simulink subsystem "Reefscape_Elevator_Motor_Control_sub"  (R2023b)
settings: Solver=VariableStepAuto  StartTime=0.0  StopTime=10.0  RelTol=1e-3
undefined symbols (not defined in the file): Elevator_Bottom_DC, Elevator_Error_Bottom_Disable, Elevator_Error_Increase, Elevator_Gain_Int, Elevator_Gain_Prop, Elevator_Height_Error_Threshold, Elevator_Height_Lower_Limit_Coral_Arm_Input, Elevator_Height_Lower_Limit_Out, Elevator_Hold_at_Top_DC, Elevator_Int_IC, Elevator_Int_LL, Elevator_Int_UL, Elevator_Total_LL, Elevator_Total_UL
libraries: simulink x6, Controls_Components_lib x1
settings Model: Creator=ander  LastModifiedBy=ander

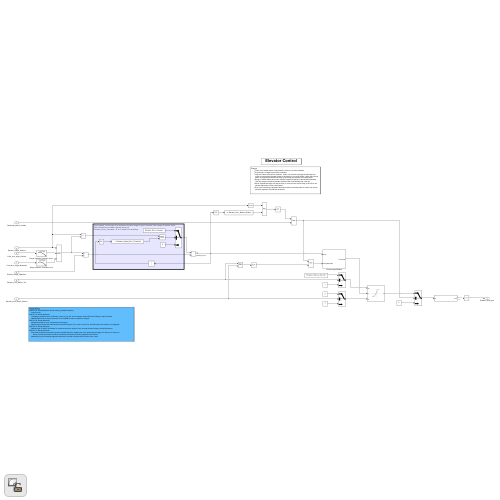
[thumbnail: Simulink's stored preview of the top-level diagram]
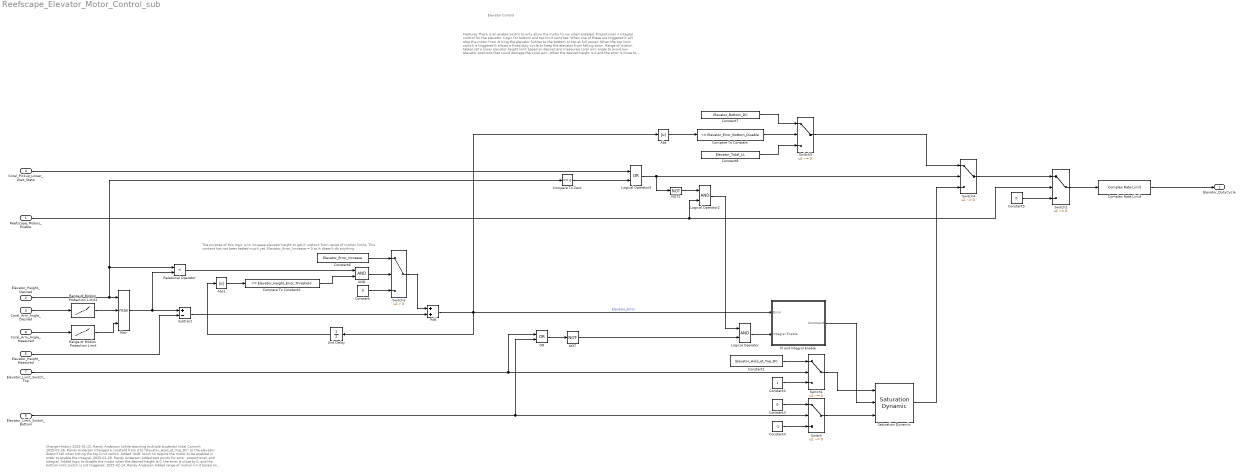
== system Reefscape_Elevator_Motor_Control_sub ==
  note: The purpose of this logic is to increase elevator height to get it unstock from range of motion limits.
      | This content has not been tested much yet.
      | Elevator_Error_Increase = 0 so it doesn't do anything.
  note: Elevator Control
  note: Features
      | There is an enable switch to only allow the motor to run when enabled.
      | Proportional + Integral control for the elevator.
      | Logic for bottom and top limit switches. When one of these are triggered it will stop the motor from driving the elevator further to the bottom or top at full power. When the top limit switch is triggered it allows a fixed duty cycle to keep the elevator from falling down.
      | Range of motion tables set a lower elevator height limit based on desired and measured coral arm angle to avoid low elevator positions that could damage the coral arm.
      | When the desired height is 0 and the error is close to 0 then set the duty cycle to 0 so the elevator falls down to hit the limit switch.
      | Duty cycle increasing magnitude rate limit provides a smoother start of motion from a stop (less jerk applied to mechanical hardware).
  note: Change History
      | 2025-01-22, Randy Anderson (while teaching multiple students)
      | Inital Commit
      | 2025-01-26, Randy Anderson
      | Changed a constant from 0 to 'Elevator_Hold_at_Top_DC' so the elevator doesn't fall when hitting the top limit switch.
      | Added 'AND' block to require the motor to be enabled in order to enable the integral.
      | 2025-01-28, Randy Anderson
      | Added test points for error, proportional, and integral.
      | Added logic to disable the motor when the desired height is 0, the error is close to 0, and the bottom limit switch is not triggered.
      | 2025-02-14, Randy Anderson
      | Added range of motion limit based on measured coral arm angle to force enough elevator height to avoid interference.
      | 2025-02-15, Randy Anderson
      | Removed the bottom limit switch input the the AND block for disabling the motor when desired height is 0 and error is close to 0.
      | When the limit switch was included it resulted in the elevator bouncing up/down off the bottom.
      | Added duty cycle increasing magnitude rate limit to provide smoother start of motion from a stop.
      | 2025-02-24, Randy Anderson
      | Added 'Coral_Pickup_Lower_Wait_State' input.
      | Added a new parameter value to force the elevator down to a fixed duty cycle in some cases.
  Reefscape_Motors_Enable : Inport
  Elevator_Height_Desired : Inport  Port=2
  Coral_Arm_Angle_Desired : Inport  Port=3
  Coral_Pickup_Lower_Wait_State : Inport  Port=4
  Elevator_Height_Measured : Inport  Port=5
  Elevator_Limit_Switch_Bottom : Inport  Port=6
  Elevator_Limit_Switch_Top : Inport  Port=7
  Coral_Arm_Angle_Measured : Inport  Port=8
  AND : Logic  AllPortsSameDT=off  OutDataTypeStr=boolean
  Abs : Abs  SaturateOnIntegerOverflow=off
  Abs1 : Abs  SaturateOnIntegerOverflow=off
  Add : Sum
  Compare To Constant : simulink/Logic and Bit Operations/Compare To Constant  relop=<=  const=Elevator_Error_Bottom_Disable  OutDataTypeStr=boolean
  Compare To Constant2 : simulink/Logic and Bit Operations/Compare To Constant  relop=<=  const=Elevator_Height_Error_Threshold  OutDataTypeStr=boolean
  Compare To Zero : simulink/Logic and Bit Operations/Compare To Zero  relop===  OutDataTypeStr=boolean
  Complex Rate Limit : Controls_Components_lib/Complex Rate Limit  Rate_Limit_Inc=Elevator_DC_Inc_RL  Rate_Limit_Dec=-1  Approaching_Zero_Error_Threshold=0.01  Approaching_Zero_Final_Scale_Factor=1  Approaching_NonZero_Error_Threshold=0.01  Approaching_NonZero_Final_Scale_Factor=1
  Constant : Constant  Value=0
  Constant1 : Constant  Value=Elevator_Hold_at_Top_DC
  Constant2 : Constant
  Constant3 : Constant  Value=0
  Constant4 : Constant  Value=-1
  Constant5 : Constant  Value=0
  Constant6 : Constant  Value=Elevator_Error_Increase
  Constant7 : Constant  Value=Elevator_Bottom_DC
  Constant8 : Constant  Value=Elevator_Total_LL
  Logical Operator : Logic  AllPortsSameDT=off  OutDataTypeStr=boolean
  Logical Operator2 : Logic  AllPortsSameDT=off  OutDataTypeStr=boolean
  Logical Operator3 : Logic  Operator=OR  AllPortsSameDT=off  OutDataTypeStr=boolean
  Max : MinMax  Function=max  Inputs=3
  NOT : Logic  Operator=NOT  AllPortsSameDT=off  OutDataTypeStr=boolean
  NOT2 : Logic  Operator=NOT  AllPortsSameDT=off  OutDataTypeStr=boolean
  OR : Logic  Operator=OR  AllPortsSameDT=off  OutDataTypeStr=boolean
  PI and Integral Enable : Subsystem  mask{Gain_P=Elevator_Gain_Prop, Gain_I=Elevator_Gain_Int, Integral_IC=Elevator_Int_IC, Limit_I_Upper=Elevator_Int_UL, Limit_I_Lower=Elevator_Int_LL, Limit_T_Upper=Elevator_Total_UL, Limit_T_Lower=Elevator_Total_LL}
      mask prompts: Gain_P "Proportional Gain"; Gain_I "Integral Gain"; Integral_IC "Integral Initial Condition"; Limit_I_Upper "Integral Upper Limit"; Limit_I_Lower "Integral Lower Limit"; Limit_T_Upper "Total Command Upper Limit"; Limit_T_Lower "Total Command Lower Limit"
  Range of Motion Protection Limit : Lookup_n-D  NumberOfTableDimensions=1  BreakpointsForDimension1=Elevator_Height_Lower_Limit_Coral_Arm_Input  Table=Elevator_Height_Lower_Limit_Out  ExtrapMethod=Clip  InternalRulePriority=Speed  RndMeth=Simplest
  Range of Motion Protection Limit1 : Lookup_n-D  NumberOfTableDimensions=1  BreakpointsForDimension1=Elevator_Height_Lower_Limit_Coral_Arm_Input  Table=Elevator_Height_Lower_Limit_Out  ExtrapMethod=Clip  InternalRulePriority=Speed  RndMeth=Simplest
  Relational Operator : RelationalOperator  Operator=<  OutDataTypeStr=boolean  RndMeth=Simplest  InputSameDT=off
  Saturation Dynamic : simulink/Discontinuities/Saturation Dynamic  OutMin=[]  OutMax=[]  OutDataTypeStr=Inherit: Same as second input  OutDataType=fixdt(1, 16)  OutScaling=2^-10  DoSatur=off
  Subtract : Sum  Inputs=+-
  Switch{,1..2,4..5} (5 alike) : Switch  Criteria=u2 ~= 0  SaturateOnIntegerOverflow=off  InputSameDT=off
  Switch3 : Switch  Criteria=u2 > Threshold  SaturateOnIntegerOverflow=off  InputSameDT=off
  Unit Delay : UnitDelay  SampleTime=-1  HasFrameUpgradeWarning=on
  Elevator_DutyCycle : Outport
  wires:
  Max/1 -> Relational Operator/2, Subtract/1
  Elevator_Limit_Switch_Bottom/1 -> Switch/2, OR/2
  PI and Integral Enable/1(Command) -> Saturation Dynamic/2
  Switch/1 -> Saturation Dynamic/3
  Switch1/1 -> Saturation Dynamic/1
  Elevator_Limit_Switch_Top/1 -> Switch1/2, OR/1
  Constant1/1 -> Switch1/1
  Constant2/1 -> Switch1/3
  Constant3/1 -> Switch/1
  Constant4/1 -> Switch/3
  OR/1 -> NOT/1
  Switch2/1 -> Complex Rate Limit/1
  Constant5/1 -> Switch2/3
  NOT/1 -> Logical Operator/2
  Logical Operator/1 -> PI and Integral Enable/2(Integral Enable)
  Elevator_Height_Measured/1 -> Subtract/2
  Subtract/1 -> Add/2
  Compare To Zero/1 -> Logical Operator3/2
  Reefscape_Motors_Enable/1 -> Switch2/2, Logical Operator2/2
  NOT2/1 -> Logical Operator2/1
  Logical Operator2/1 -> Logical Operator/1
  Complex Rate Limit/1 -> Elevator_DutyCycle/1
  Coral_Arm_Angle_Measured/1 -> Range of Motion Protection Limit/1
  Range of Motion Protection Limit/1 -> Max/3
  Elevator_Height_Desired/1 -> Max/1, Compare To Zero/1, Relational Operator/1
  Range of Motion Protection Limit1/1 -> Max/2
  Coral_Arm_Angle_Desired/1 -> Range of Motion Protection Limit1/1
  Compare To Constant2/1 -> AND/2
  Abs1/1 -> Compare To Constant2/1
  Relational Operator/1 -> AND/1
  AND/1 -> Switch3/2
  Constant/1 -> Switch3/3
  Switch3/1 -> Add/1
  Add/1 -> PI and Integral Enable/1(Error), Unit Delay/1, Abs/1  "Elevator_Error"
  Constant6/1 -> Switch3/1
  Unit Delay/1 -> Abs1/1
  Saturation Dynamic/1 -> Switch4/3
  Switch4/1 -> Switch2/1
  Logical Operator3/1 -> NOT2/1, Switch4/2
  Coral_Pickup_Lower_Wait_State/1 -> Logical Operator3/1
  Switch5/1 -> Switch4/1
  Constant7/1 -> Switch5/1
  Compare To Constant/1 -> Switch5/2
  Abs/1 -> Compare To Constant/1
  Constant8/1 -> Switch5/3

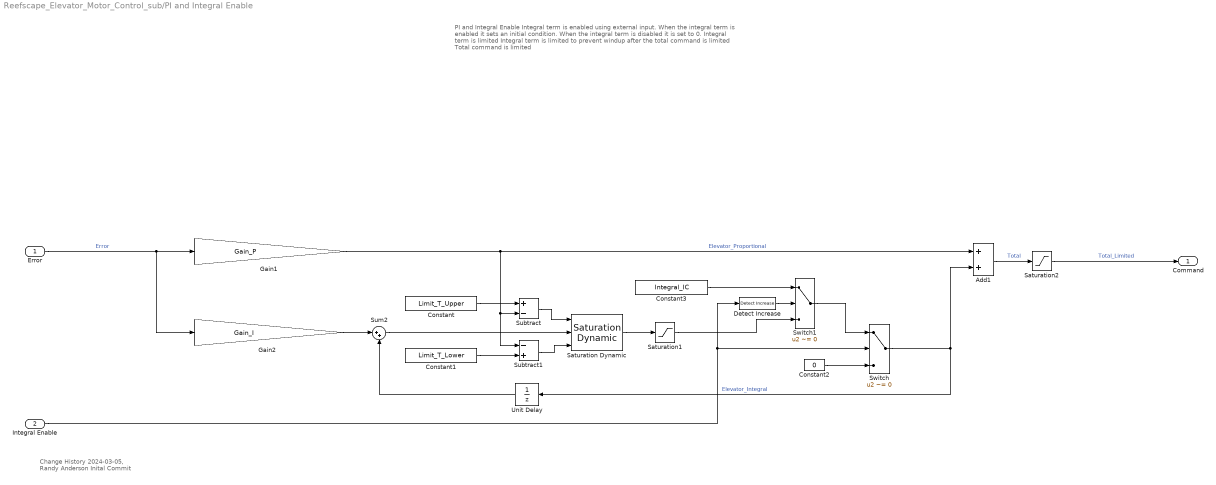
== system Reefscape_Elevator_Motor_Control_sub/PI and Integral Enable ==
  note: PI and Integral Enable
      |
      | Integral term is enabled using external input.
      | When the integral term is enabled it sets an initial condition.
      | When the integral term is disabled it is set to 0.
      |
      | Integral term is limited
      |
      | Integral term is limited to prevent windup after the total command is limited
      |
      | Total command is limited
  note: Change History
      | 2024-03-05, Randy Anderson
      | Inital Commit
  Error : Inport
  Integral Enable : Inport  Port=2
  Add1 : Sum  Inputs=2
  Constant : Constant  Value=Limit_T_Upper
  Constant1 : Constant  Value=Limit_T_Lower
  Constant2 : Constant  Value=0
  Constant3 : Constant  Value=Integral_IC
  Detect Increase : simulink/Logic and Bit Operations/Detect Increase  vinit=0.0  OutDataTypeStr=boolean
  Gain1 : Gain  Gain=Gain_P
  Gain2 : Gain  Gain=Gain_I
  Saturation Dynamic : simulink/Discontinuities/Saturation Dynamic  OutMin=[]  OutMax=[]  OutDataTypeStr=Inherit: Same as second input  OutDataType=fixdt(1, 16)  OutScaling=2^-10  DoSatur=off
  Saturation1 : Saturate  UpperLimit=Limit_I_Upper  LowerLimit=Limit_I_Lower
  Saturation2 : Saturate  UpperLimit=Limit_T_Upper  LowerLimit=Limit_T_Lower
  Subtract : Sum  Inputs=+-
  Subtract1 : Sum  Inputs=-+
  Sum2 : Sum  Inputs=|++
  Switch : Switch  Criteria=u2 ~= 0  SaturateOnIntegerOverflow=off  InputSameDT=off
  Switch1 : Switch  Criteria=u2 ~= 0  SaturateOnIntegerOverflow=off  InputSameDT=off
  Unit Delay : UnitDelay  SampleTime=-1  HasFrameUpgradeWarning=on
  Command : Outport
  wires:
  Constant2/1 -> Switch/3
  Integral Enable/1 -> Detect Increase/1, Switch/2
  Error/1 -> Gain2/1, Gain1/1  "Error"
  Subtract1/1 -> Saturation Dynamic/3
  Gain1/1 -> Add1/1, Subtract1/1, Subtract/2  "Elevator_Proportional"
  Gain2/1 -> Sum2/1
  Saturation Dynamic/1 -> Saturation1/1
  Subtract/1 -> Saturation Dynamic/1
  Unit Delay/1 -> Sum2/2
  Constant/1 -> Subtract/1
  Constant1/1 -> Subtract1/2
  Add1/1 -> Saturation2/1  "Total"
  Sum2/1 -> Saturation Dynamic/2
  Saturation2/1 -> Command/1  "Total_Limited"
  Switch/1 -> Unit Delay/1, Add1/2  "Elevator_Integral"
  Switch1/1 -> Switch/1
  Detect Increase/1 -> Switch1/2
  Saturation1/1 -> Switch1/3
  Constant3/1 -> Switch1/1
